simulink model "Problem2"  (R2020b)
settings: Solver=VariableStepAuto  StartTime=0.0  StopTime=10.0  RelTol=1e-3
model workspace (MAT data in the model file):
  M1 = Simulink.Parameter
  M1.Value = 2500
  M1.DataType = 'auto'
  M1.Dimensions = [1 1]
  M2 = Simulink.Parameter
  M2.Value = 320
  M2.DataType = 'auto'
  M2.Dimensions = [1 1]
  b = Simulink.Parameter
  b.Value = 350
  b.DataType = 'auto'
  b.Dimensions = [1 1]
  k1 = Simulink.Parameter
  k1.Value = 80000
  k1.DataType = 'auto'
  k1.Dimensions = [1 1]
  k2 = Simulink.Parameter
  k2.Value = 500000
  k2.DataType = 'auto'
  k2.Dimensions = [1 1]
settings Model: Creator=ASUS  LastModifiedBy=ASUS

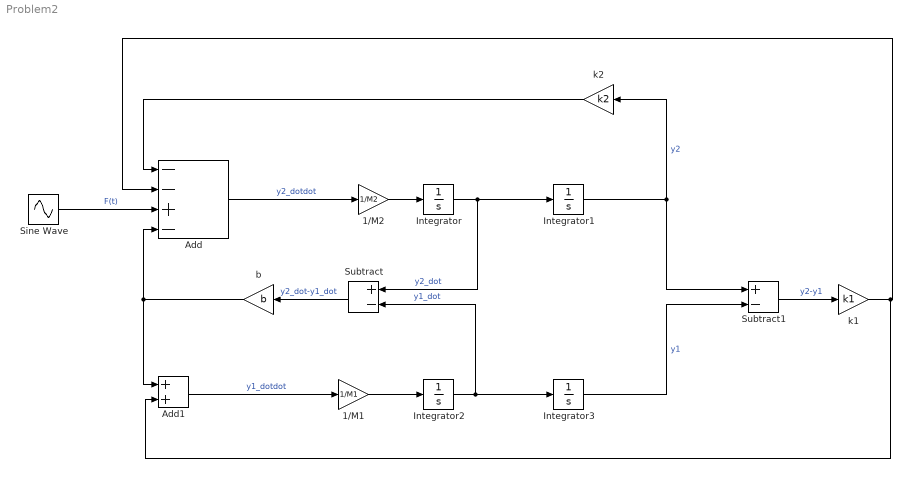
== system Problem2 ==
  1/M1 : Gain  Gain=1/M1
  1/M2 : Gain  Gain=1/M2
  Add : Sum  Inputs=--+-
  Add1 : Sum
  Integrator{,1..3} (4 alike) : Integrator
  Sine Wave : Sin  SampleTime=0
  Subtract : Sum  Inputs=+-
  Subtract1 : Sum  Inputs=+-
  b : Gain  Gain=b
  k1 : Gain  Gain=k1
  k2 : Gain  Gain=k2
  wires:
  Add/1 -> 1/M2/1  "y2_dotdot"
  1/M2/1 -> Integrator/1
  Integrator/1 -> Integrator1/1, Subtract/1  "y2_dot"
  Integrator1/1 -> k2/1, Subtract1/1  "y2"
  Sine Wave/1 -> Add/3  "F(t)"
  Add1/1 -> 1/M1/1  "y1_dotdot"
  1/M1/1 -> Integrator2/1
  Integrator2/1 -> Subtract/2, Integrator3/1  "y1_dot"
  Integrator3/1 -> Subtract1/2  "y1"
  Subtract/1 -> b/1  "y2_dot-y1_dot"
  Subtract1/1 -> k1/1  "y2-y1"
  k1/1 -> Add1/2, Add/2
  k2/1 -> Add/1
  b/1 -> Add1/1, Add/4
